simulink model "DRISHTI_Screening_System"  (R2026a)
settings: Solver=FixedStepAuto  StopTime=1
undefined symbols (not defined in the file or in its folder): DRISHTI_gradeInput, DRISHTI_modelScore, DRISHTI_qualityScore
libraries: simulink x1
Description:
  | DRISHTI - Explainable AI for Diabetic Retinopathy Screening
  | System-level MATLAB/Simulink model for rural screening workflow.
  | MATLAB performs AI algorithms; Simulink models workflow, decisions,
  | timing, throughput and human-in-the-loop behavior.
settings Model: Creator=SHIVANYA SALES  LastModifiedBy=SHIVANYA SALES

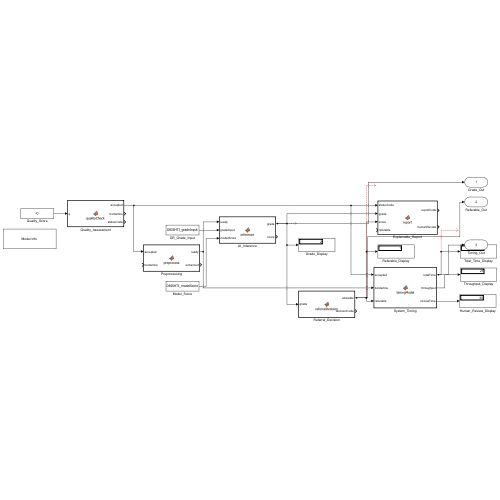
[thumbnail: Simulink's stored preview of the top-level diagram]
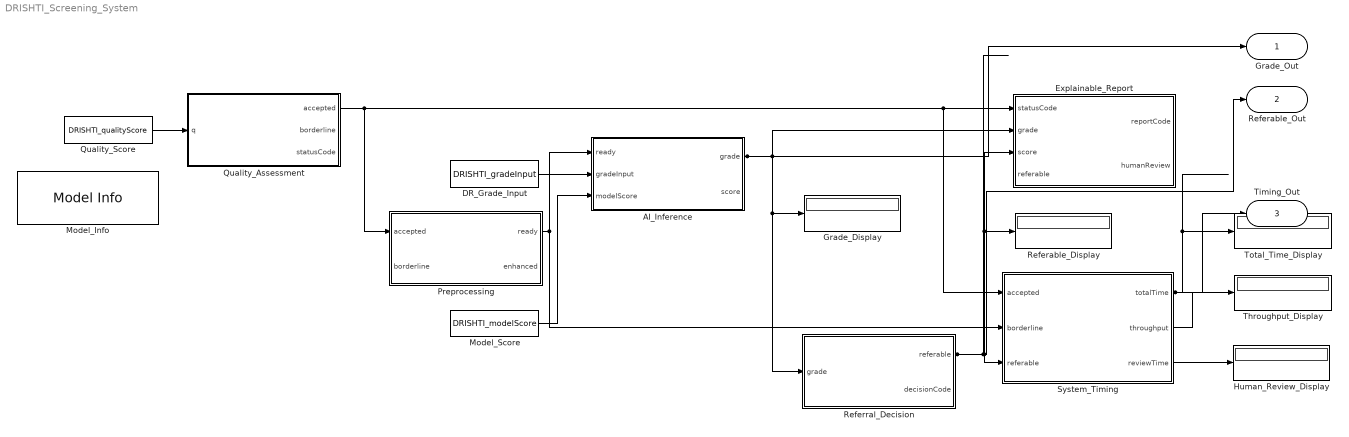
== system DRISHTI_Screening_System ==
  AI_Inference : MATLAB Function  TreatAsAtomicUnit=on
  DR_Grade_Input : Constant  Value=DRISHTI_gradeInput
  Explainable_Report : MATLAB Function  TreatAsAtomicUnit=on
  Grade_Display : Display
  Human_Review_Display : Display
  Model_Info : simulink/Model-Wide Utilities/Model Info  Frame=on  DisplayStringWithTags=Model Info  HorizontalTextAlignment=Center  LeftAlignmentValue=0.5
  Model_Score : Constant  Value=DRISHTI_modelScore
  Preprocessing : MATLAB Function  TreatAsAtomicUnit=on
  Quality_Assessment : MATLAB Function  TreatAsAtomicUnit=on
  Quality_Score : Constant  Value=DRISHTI_qualityScore
  Referable_Display : Display
  Referral_Decision : MATLAB Function  TreatAsAtomicUnit=on
  System_Timing : MATLAB Function  TreatAsAtomicUnit=on
  Throughput_Display : Display
  Total_Time_Display : Display
  Grade_Out : Outport
  Referable_Out : Outport  Port=2
  Timing_Out : Outport  Port=3
  wires:
  System_Timing/1(totalTime) -> Total_Time_Display/1, Timing_Out/1
  Quality_Score/1 -> Quality_Assessment/1(q)
  Model_Score/1 -> AI_Inference/3(modelScore)
  DR_Grade_Input/1 -> AI_Inference/2(gradeInput)
  Quality_Assessment/1(accepted) -> Explainable_Report/1(statusCode), System_Timing/1(accepted), Preprocessing/1(accepted)
  Preprocessing/1(ready) -> System_Timing/2(borderline), AI_Inference/1(ready)
  AI_Inference/1(grade) -> Grade_Display/1, Referral_Decision/1(grade), Explainable_Report/2(grade), Grade_Out/1
  System_Timing/3(reviewTime) -> Human_Review_Display/1
  Referral_Decision/1(referable) -> Referable_Display/1, Explainable_Report/3(score), System_Timing/3(referable), Referable_Out/1
  System_Timing/2(throughput) -> Throughput_Display/1

== matlab function DRISHTI_Screening_System/Preprocessing ==
  data: accepted input double size=[1 1]; ready output double size=[1 1]; borderline input double size=[1 1]; enhanced output double size=[1 1]
function [ready,enhanced] = preprocess(accepted,borderline)

% Force scalar inputs
accepted   = accepted(1);
borderline = borderline(1);

% Explicit scalar outputs
ready    = 0.0;
enhanced = 0.0;

if accepted == 0

    ready = 0.0;
    enhanced = 0.0;

elseif borderline ~= 0

    ready = 1.0;
    enhanced = 1.0;

else

    ready = 1.0;
    enhanced = 0.0;

end

end

== matlab function DRISHTI_Screening_System/Quality_Assessment ==
  data: q input double size=[1 1]; accepted output double size=[1 1]; borderline output double size=[1 1]; statusCode output double size=[1 1]
function [accepted,borderline,statusCode] = qualityCheck(q)

% Force scalar input
q = q(1);

% Explicit scalar outputs
accepted   = 0.0;
borderline = 0.0;
statusCode = 0.0;

if q < 0.40

    % REJECT
    accepted   = 0.0;
    borderline = 0.0;
    statusCode = 0.0;

elseif q < 0.65

    % BORDERLINE
    accepted   = 1.0;
    borderline = 1.0;
    statusCode = 1.0;

else

    % ACCEPT
    accepted   = 1.0;
    borderline = 0.0;
    statusCode = 2.0;

end

end

== matlab function DRISHTI_Screening_System/AI_Inference ==
  data: ready input double size=[1 1]; grade output double size=[1 1]; gradeInput input double size=[1 1]; modelScore input double size=[1 1]; score output double size=[1 1]
function [grade,score] = inference(ready,gradeInput,modelScore)

ready      = ready(1);
gradeInput = gradeInput(1);
modelScore = modelScore(1);

grade = -1.0;
score = 0.0;

if ready ~= 0

    grade = gradeInput;
    score = modelScore;

end

end

== matlab function DRISHTI_Screening_System/Referral_Decision ==
  data: grade input double size=[1 1]; referable output double size=[1 1]; decisionCode output double size=[1 1]
function [referable,decisionCode] = referralDecision(grade)

grade = grade(1);

referable   = 0.0;
decisionCode = 0.0;

if grade < 0

    referable = 0.0;
    decisionCode = 0.0;

elseif grade >= 2

    referable = 1.0;
    decisionCode = 2.0;

else

    referable = 0.0;
    decisionCode = 1.0;

end

end

== matlab function DRISHTI_Screening_System/Explainable_Report ==
  data: statusCode input double size=[1 1]; reportCode output double size=[1 1]; grade input double size=[1 1]; score input double size=[1 1]; referable input double size=[1 1]; humanReview output double size=[1 1]
function [reportCode,humanReview] = report( ...
    statusCode,grade,score,referable)

statusCode = statusCode(1);
grade      = grade(1);
score      = score(1);
referable  = referable(1);

reportCode = 0.0;
humanReview = 0.0;

if statusCode == 0

    % Rejected image
    reportCode = 0.0;
    humanReview = 0.0;

elseif grade >= 2 && referable ~= 0

    % Referable DR
    reportCode = 2.0;
    humanReview = 1.0;

else

    % Non-referable
    reportCode = 1.0;
    humanReview = 0.0;

end

end

== matlab function DRISHTI_Screening_System/System_Timing ==
  data: accepted input size=[1 1]; totalTime output size=[1 1]; borderline input size=[1 1]; referable input size=[1 1]; throughput output size=[1 1]; reviewTime output size=[1 1]
function [totalTime,throughput,reviewTime] = timingModel( ...
    accepted,borderline,referable)

% Force all inputs to scalar values
accepted   = accepted(1);
borderline = borderline(1);
referable  = referable(1);

% Engineering timing assumptions
qualityTime    = 0.20;
preprocessTime = 0.30;
inferenceTime  = 1.00;
explainTime    = 0.50;
reportTime     = 0.20;
humanTime      = 30.0;

% Initialize scalar outputs explicitly
totalTime  = 0.0;
throughput = 0.0;
reviewTime = 0.0;

% Screening timing
if ~accepted

    totalTime = qualityTime;

else

    totalTime = ...
        qualityTime + ...
        preprocessTime + ...
        inferenceTime + ...
        explainTime + ...
        reportTime;

    % Additional processing for borderline images
    if borderline
        totalTime = totalTime + 0.20;
    end

    % Human-in-the-loop review
    if referable
        reviewTime = humanTime;
    end

end

% Automated throughput
throughput = 60.0 / totalTime;

end
